simulink model "poleplacemente_ciclochiuso_WP2"  (R2023a)
settings: Solver=VariableStepAuto  StartTime=0.0  StopTime=10.0  RelTol=1e-3
values from neighbouring files (symbols this model uses):
  K = [k1 k2]    [WP2.m]    (also in parameters_for_equipollenza_WP2.m = [8109.81 179.9]; poleplacement_WP2.m = [1609.81 39.90]; poleplacement_test1_WP2.m = [739.81 53.9]; poleplacement_test2_WP2.m = [17.1 5.3])
  k_r = -1/(C*inv(A-B*K)*B)    [poleplacement_WP2.m]    (also in poleplacement_test1_WP2.m; poleplacement_test2_WP2.m; poleplacement_test3_WP2.m; poleplacement_test4_WP2.m)
settings Model: Creator=miche  LastModifiedBy=miche

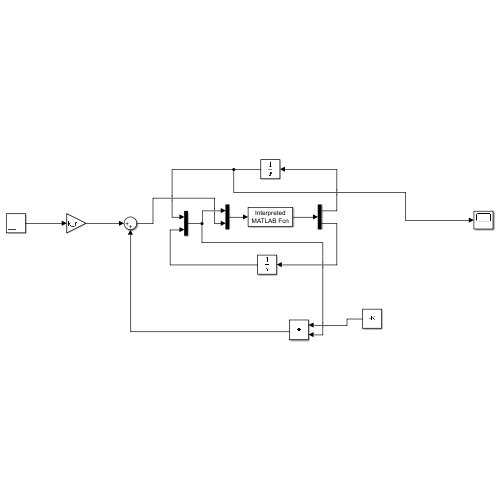
[thumbnail: Simulink's stored preview of the top-level diagram]
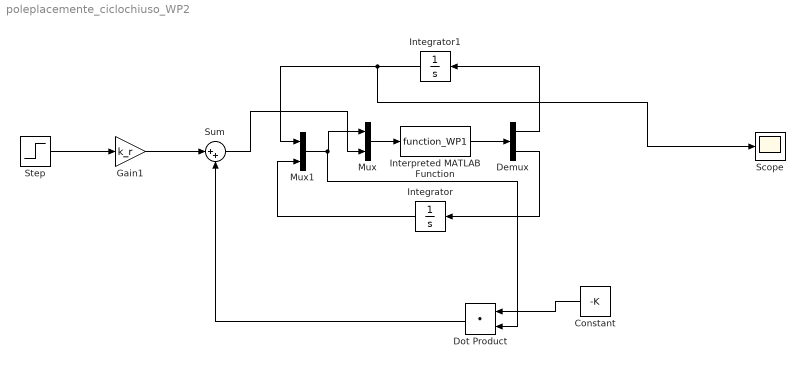
== system poleplacemente_ciclochiuso_WP2 ==
  Constant : Constant  Value=-K
  Demux : Demux  Outputs=2
  Dot Product : DotProduct  OutDataTypeStr=Inherit: Inherit via internal rule
  Gain1 : Gain  Gain=k_r
  Integrator : Integrator
  Integrator1 : Integrator
  Interpreted MATLAB Function : MATLABFcn  MATLABFcn=function_WP1  OutputDimensions=2
  Mux : Mux  Inputs=2
  Mux1 : Mux  Inputs=2
  Scope : Scope
  Step : Step  After=pi  SampleTime=0
  Sum : Sum  Inputs=|++
  wires:
  Mux1/1 -> Dot Product/2, Mux/1
  Integrator1/1 -> Scope/1, Mux1/1
  Interpreted MATLAB Function/1 -> Demux/1
  Demux/2 -> Integrator/1
  Demux/1 -> Integrator1/1
  Mux/1 -> Interpreted MATLAB Function/1
  Integrator/1 -> Mux1/2
  Sum/1 -> Mux/2
  Step/1 -> Gain1/1
  Gain1/1 -> Sum/1
  Constant/1 -> Dot Product/1
  Dot Product/1 -> Sum/2
